simulink model "QD2_DroneStack_PID_FreqSwp_2021a"  (R2026a)
settings: Solver=ode1  StopTime=inf  FixedStep=1/1000  EnableMultiTasking=on
InitFcn:
  | Motor_Mapping_7_Inch
model workspace (MAT data in the model file):
  target_system = 1
undefined symbols (not defined in the file): _Commander, _Stabilizer, _SYSID, datetime, HIL, KT, lf, log_, log_QD2_, m, Motor_Matrix, n, qc_get_step_size, s, saved_data
libraries: quarc_library x107, simulink x30, simulink_extras x3, sl_discontinuities x2
(part 3 of 5)

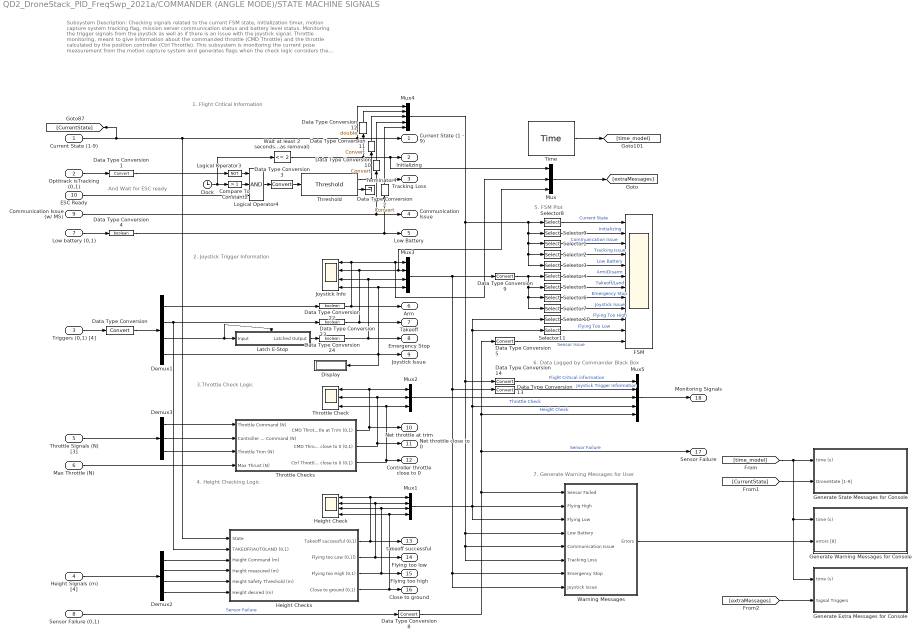
== system QD2_DroneStack_PID_FreqSwp_2021a/COMMANDER (ANGLE MODE)/STATE MACHINE SIGNALS ==
  note: 4. Height Checking Logic
  note: 3.Throttle Check Logic
  note: 2. Joystick Trigger Information
  note: 1. Flight Critical Information
  note: 6. Data Logged by Commander Black Box
  note: 5. FSM Plot
  note: 7. Generate Warning Messages for User
  note: Subsystem Description:
      | Checking signals related to the current FSM state, initialization timer, motion capture system tracking flag, mission server communication status and battery level status.
      | Monitoring the trigger signals from the joystick as well as if there is an issue with the joystick signal.
      | Throttle monitoring, meant to give information about the commanded throttle (CMD Throttle) and the throttle calculated by the position controller (Ctrl Throttle).
      | This subsystem is monitoring the current pose measurement from the motion capture system and generates flags when the check logic considers the QDrone flying to close to ground, too high or too low as well as generate a successful take off flag.
      | A subset of the FSM monitoring signals are shown using this scope. These signals are what Quanser considers importnat for flight.
      | FSM signals sent to the blackbox for post flight monitoring.
      | Error message generation based on flags generated by the FSM signal checks.
  note: And Wait for ESC ready
  Current State (1-9) : Inport
  "Optitrack isTracking (0,1)  " : Inport  Port=2
  Triggers (0,1) [4] : Inport  Port=3
  Height Signals (m) [4] : Inport  Port=4
  Throttle Signals (N) [3] : Inport  Port=5
  "Max Throttle (N) " : Inport  Port=6
  Low battery (0,1) : Inport  Port=7
  Sensor Failure (0,1) : Inport  Port=8
  Communication Issue (w/ MS) : Inport  Port=9
  ESC Ready : Inport  Port=10
  Clock : Clock
  Compare To Constant2 : simulink/Logic and Bit Operations/Compare To Constant  relop=>  const=1  OutDataTypeStr=boolean
  Data Type Conversion{,1..3,5,8..11,13..14} (11 alike) : DataTypeConversion  SaturateOnIntegerOverflow=off  RndMeth=Floor
  Data Type Conversion12 : DataTypeConversion  OutDataTypeStr=double  SaturateOnIntegerOverflow=off  RndMeth=Floor
  Data Type Conversion{4,22..24} (4 alike) : DataTypeConversion  OutDataTypeStr=boolean  SaturateOnIntegerOverflow=off  RndMeth=Floor
  Demux1 : Demux  Outputs=[1 1 1 1]
  Demux2 : Demux
  Demux3 : Demux  Outputs=3
  Display : Display
  FSM : Scope  NumInputPorts=12
      settings: TimeSpan=30  Title=Current State  ActiveDisplayYMinimum=0.9  ActiveDisplayYMaximum=1.1
  Generate Extra Messages for Console : Subsystem
  Generate State Messages for Console : Subsystem
  Generate Warning Messages for Console : Subsystem
  "Height Check " : Scope  NumInputPorts=4
      settings: Title=Takeoff Successful  ActiveDisplayYMinimum=-1  ActiveDisplayYMaximum=1  DataLoggingVariableName=ScopeData3
  Height Checks : Subsystem
  Joystick Info : Scope  NumInputPorts=4
      settings: Title=Arm
  Latch E-Stop : Subsystem  TreatAsAtomicUnit=on
  Logical Operator3 : Logic  Operator=NOT  AllPortsSameDT=off  OutDataTypeStr=boolean
  Logical Operator4 : Logic  Inputs=3  AllPortsSameDT=off  OutDataTypeStr=boolean
  Mux : Mux  Inputs=3
  Mux1 : Mux  Inputs=[1 1 1 1]
  Mux2 : Mux  Inputs=[1 1 1]
  Mux3 : Mux  Inputs=[1 1 1 1]
  Mux4 : Mux  Inputs=[1 1 1 1 1]
  Mux5 : Mux  Inputs=[5 4 3 4 1]
  Selector1 : Selector  InputPortWidth=5  IndexOptions=Index vector (dialog)  Indices=4  OutputSizes=1
  Selector10 : Selector  InputPortWidth=4  IndexOptions=Index vector (dialog)  Indices=3  OutputSizes=1
  Selector11 : Selector  InputPortWidth=4  IndexOptions=Index vector (dialog)  Indices=2  OutputSizes=1
  Selector2 : Selector  InputPortWidth=5  IndexOptions=Index vector (dialog)  Indices=3  OutputSizes=1
  Selector3 : Selector  InputPortWidth=5  IndexOptions=Index vector (dialog)  Indices=5  OutputSizes=1
  Selector4 : Selector  InputPortWidth=4  IndexOptions=Index vector (dialog)  Indices=1  OutputSizes=1
  Selector5 : Selector  InputPortWidth=4  IndexOptions=Index vector (dialog)  Indices=2  OutputSizes=1
  Selector6 : Selector  InputPortWidth=4  IndexOptions=Index vector (dialog)  Indices=3  OutputSizes=1
  Selector7 : Selector  InputPortWidth=4  IndexOptions=Index vector (dialog)  Indices=4  OutputSizes=1
  Selector8 : Selector  InputPortWidth=5  IndexOptions=Index vector (dialog)  Indices=1  OutputSizes=1
  Selector9 : Selector  InputPortWidth=5  IndexOptions=Index vector (dialog)  Indices=2  OutputSizes=1
  Terminator4 : Terminator
  Threshold : quarc_library/Discontinuities/Threshold  operator=>=  param_src=Specify via dialog  threshold=0.5  duration=0.2
      settings: SourceProductName=QUARC Targets
  Throttle Check : Scope  NumInputPorts=3
      settings: Title=Command Throttle At Trim  ActiveDisplayYMinimum=-0.125  ActiveDisplayYMaximum=1.125  DataLoggingVariableName=ScopeData2
  Throttle Checks : Subsystem
  Time : quarc_library/Sources/Time/Time  time_source=Wall clock  sample_time=qc_get_step_size
  "Wait at least 2 seconds to allow for initialization (e.g., bias removal)" : simulink/Logic and Bit Operations/Compare To Constant  relop=<=  const=2  OutDataTypeStr=boolean
  Warning Messages : Subsystem
  "Current State (1 - 9)  " : Outport  VectorParamsAs1DForOutWhenUnconnected=off
  Initializing : Outport  Port=2  VectorParamsAs1DForOutWhenUnconnected=off
  Tracking Loss : Outport  Port=3  VectorParamsAs1DForOutWhenUnconnected=off
  Communication Issue : Outport  Port=4  VectorParamsAs1DForOutWhenUnconnected=off
  Low Battery : Outport  Port=5  VectorParamsAs1DForOutWhenUnconnected=off
  Arm : Outport  Port=6  VectorParamsAs1DForOutWhenUnconnected=off
  Takeoff : Outport  Port=7  VectorParamsAs1DForOutWhenUnconnected=off
  Emergency Stop : Outport  Port=8  VectorParamsAs1DForOutWhenUnconnected=off
  "Joystick Issue " : Outport  Port=9  VectorParamsAs1DForOutWhenUnconnected=off
  Net throttle at trim : Outport  Port=10  VectorParamsAs1DForOutWhenUnconnected=off
  Net throttle close to 0 : Outport  Port=11  VectorParamsAs1DForOutWhenUnconnected=off
  Controller throttle close to 0 : Outport  Port=12  VectorParamsAs1DForOutWhenUnconnected=off
  takeoff successful : Outport  Port=13  VectorParamsAs1DForOutWhenUnconnected=off
  Flying too low : Outport  Port=14  VectorParamsAs1DForOutWhenUnconnected=off
  Flying too high : Outport  Port=15  VectorParamsAs1DForOutWhenUnconnected=off
  Close to ground : Outport  Port=16  VectorParamsAs1DForOutWhenUnconnected=off
  "  Sensor Failure" : Outport  Port=17  VectorParamsAs1DForOutWhenUnconnected=off
  Monitoring Signals : Outport  Port=18  VectorParamsAs1DForOutWhenUnconnected=off
  wires:
  ESC Ready/1 -> Logical Operator4/3
  [extraMessages] -> Generate Extra Messages for Console/2(Signal Triggers)
  Mux/1 -> [extraMessages]
  Warning Messages/1(Errors) -> Generate Warning Messages for Console/2(errors [8])
  [CurrentState] -> Generate State Messages for Console/2(DroneState [1-9])
  [time_model] -> Generate State Messages for Console/1(time (s)), Generate Extra Messages for Console/1(time (s)), Generate Warning Messages for Console/1(time (s))
  Time/1 -> [time_model]
  "Max Throttle (N) "/1 -> Throttle Checks/4(Max Thrust (N))
  "Wait at least 2 seconds to allow for initialization (e.g., bias removal)"/1 -> Initializing/1, Mux/1, Data Type Conversion12/1
  Data Type Conversion14/1 -> Mux5/1  "Flight Critical information"
  Data Type Conversion13/1 -> Mux5/2  "Joystick Trigger Information"
  Data Type Conversion12/1 -> Mux4/2
  Data Type Conversion11/1 -> Mux4/3
  Data Type Conversion10/1 -> Mux4/4
  Data Type Conversion2/1 -> Mux4/5
  Selector8/1 -> FSM/1  "Current State"
  Current State (1-9)/1 -> "Current State (1 - 9)  "/1, Mux4/1, Height Checks/1(State), [CurrentState]
  Data Type Conversion8/1 -> Warning Messages/1(Sensor Failed), Mux5/5, Data Type Conversion5/1, "  Sensor Failure"/1  "Sensor Failure"
  Data Type Conversion9/1 -> Selector6/1, Selector7/1, Selector5/1, Selector4/1
  Throttle Checks/3(Ctrl Throttle close to 0 (0,1)) -> Controller throttle close to 0/1, Throttle Check/3, Mux2/3
  Mux4/1 -> Selector8/1, Selector9/1, Selector1/1, Selector2/1, Selector3/1, Data Type Conversion14/1, Warning Messages/6(Tracking Loss), Warning Messages/5(Communication Issue), Warning Messages/4(Low Battery)
  Mux3/1 -> Data Type Conversion13/1, Warning Messages/8(Joystick Issue), Warning Messages/7("Emergency Stop "), Data Type Conversion9/1
  Mux2/1 -> Mux5/3  "Throttle Check"
  Mux1/1 -> Mux5/4, Selector10/1, Selector11/1, Warning Messages/2(Flying High), Warning Messages/3(Flying Low)  "Height Check"
  Mux5/1 -> Monitoring Signals/1
  Threshold/1 -> Tracking Loss/1, Data Type Conversion11/1
  Communication Issue (w/ MS)/1 -> Communication Issue/1, Data Type Conversion10/1
  Demux1/4 -> "Joystick Issue "/1, Mux3/4, Joystick Info/4, Display/1
  Data Type Conversion4/1 -> Low Battery/1, Data Type Conversion2/1
  Data Type Conversion22/1 -> Arm/1, Mux3/1, Mux/2, Joystick Info/1
  Data Type Conversion23/1 -> Takeoff/1, Mux3/2, Mux/3, Joystick Info/2
  Data Type Conversion24/1 -> Emergency Stop/1, Mux3/3, Joystick Info/3
  Selector11/1 -> FSM/11  "Flying Too Low"
  Selector10/1 -> FSM/10  "Flying Too High"
  Data Type Conversion5/1 -> FSM/12  "Sensor Issue"
  Selector7/1 -> FSM/9  "Joystick Issue"
  Selector6/1 -> FSM/8  "Emergency Stop"
  Selector5/1 -> FSM/7  "Takeoff/Land"
  Selector4/1 -> FSM/6  "Arm/Disarm"
  Selector3/1 -> FSM/5  "Low Battery"
  Selector2/1 -> FSM/4  "Tracking Issue"
  Selector1/1 -> FSM/3  "Communication Issue"
  Selector9/1 -> FSM/2  "Initializing"
  Demux1/3 -> Latch E-Stop/Trigger, Latch E-Stop/1(Input)
  Latch E-Stop/1(Latched Output) -> Data Type Conversion24/1
  "Optitrack isTracking (0,1)  "/1 -> Data Type Conversion1/1
  Logical Operator3/1 -> Logical Operator4/1
  Threshold/2 -> Terminator4/1
  Logical Operator4/1 -> Data Type Conversion3/1
  Clock/1 -> Compare To Constant2/1, "Wait at least 2 seconds to allow for initialization (e.g., bias removal)"/1
  Compare To Constant2/1 -> Logical Operator4/2
  Data Type Conversion3/1 -> Threshold/1
  Data Type Conversion1/1 -> Logical Operator3/1
  Sensor Failure (0,1)/1 -> Data Type Conversion8/1  "Sensor Failure"
  Height Checks/2(Flying too Low (0,1l)) -> "Height Check "/2, Mux1/2, Flying too low/1
  Low battery (0,1)/1 -> Data Type Conversion4/1
  Data Type Conversion/1 -> Demux1/1
  Height Checks/4(Close to ground (0,1)) -> Close to ground/1, Mux1/4, "Height Check "/4
  Height Checks/3(Flying too High (0,1)) -> Flying too high/1, "Height Check "/3, Mux1/3
  Throttle Checks/1(CMD Throttle at Trim (0,1)) -> Throttle Check/1, Mux2/1, Net throttle at trim/1
  Demux3/3 -> Throttle Checks/3(Throttle Trim (N))
  Demux3/2 -> Throttle Checks/2(Controller Throttle Command (N))
  Demux2/2 -> Height Checks/4(Height measured (m))
  Demux1/2 -> Height Checks/2(TAKEOFF/AUTOLAND (0,1)), Data Type Conversion23/1
  Demux2/3 -> Height Checks/5(Height Safety Threshold (m))
  Height Checks/1(Takeoff successful (0,1)) -> Mux1/1, "Height Check "/1, takeoff successful/1
  Throttle Checks/2(CMD Throttle close to 0 (0,1)) -> Net throttle close to 0/1, Throttle Check/2, Mux2/2
  Demux1/1 -> Data Type Conversion22/1
  Throttle Signals (N) [3]/1 -> Demux3/1
  Demux2/4 -> Height Checks/6(Height desired (m))
  Height Signals (m) [4]/1 -> Demux2/1
  Demux3/1 -> Throttle Checks/1(Throttle Command (N))
  Demux2/1 -> Height Checks/3(Height Command (m))
  Triggers (0,1) [4]/1 -> Data Type Conversion/1

== system QD2_DroneStack_PID_FreqSwp_2021a/COMMANDER (ANGLE MODE)/Signal Smoothing ==
  "High Frequency Controller Commands (N,rad, rad/s)[4]" : Inport
  Constant4 : Constant
  Constant5 : Constant  Value=100
  Mux : Mux  Inputs=2
  Second-Order Low-Pass Filter : quarc_library/Continuous/Second-Order Low-Pass Filter  params_source=External (input ports)  input_width=60  input_zeta=1  input_init=0
  Selector1 : Selector  InputPortWidth=4  IndexOptions=Index vector (dialog)  Indices=[3:4]  OutputSizes=1
  Selector3 : Selector  InputPortWidth=4  IndexOptions=Index vector (dialog)  Indices=[1:2]  OutputSizes=1
  Terminator : Terminator
  "Smoothed Controller Commands (N,rad, rad/s)[4]" : Outport
  wires:
  Second-Order Low-Pass Filter/2 -> Terminator/1
  Constant5/1 -> Second-Order Low-Pass Filter/2
  Constant4/1 -> Second-Order Low-Pass Filter/3
  Selector3/1 -> Second-Order Low-Pass Filter/1, Second-Order Low-Pass Filter/4
  Second-Order Low-Pass Filter/1 -> Mux/1
  Selector1/1 -> Mux/2
  Mux/1 -> "Smoothed Controller Commands (N,rad, rad/s)[4]"/1
  "High Frequency Controller Commands (N,rad, rad/s)[4]"/1 -> Selector3/1, Selector1/1

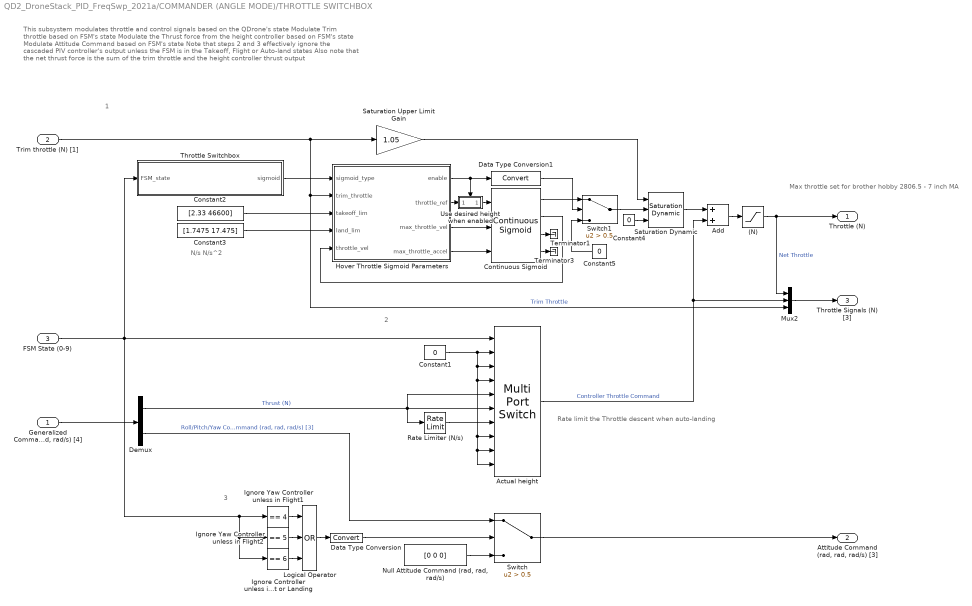
== system QD2_DroneStack_PID_FreqSwp_2021a/COMMANDER (ANGLE MODE)/THROTTLE SWITCHBOX  ==
  note: N/s N/s^2
  note: This subsystem modulates throttle and control signals based on the QDrone's state
      | Modulate Trim throttle based on FSM's state
      | Modulate the Thrust force from the height controller based on FSM's state
      | Modulate Attitude Command based on FSM's state
      |
      | Note that steps 2 and 3 effectively ignore the cascaded PIV controller's output unless the FSM is in the Takeoff, Flight or Auto-land states
      | Also note that the net thrust force is the sum of the trim throttle and the height controller thrust output
  note: Rate limit the Throttle descent when auto-landing
  note: 1
  note: 2
  note: 3
  note: Max throttle set for brother hobby 2806.5 - 7 inch MA
  "Generalized Command (N, rad, rad, rad/s) [4]" : Inport
  Trim throttle (N) [1] : Inport  Port=2
  FSM State (0-9) : Inport  Port=3
  (N) : Saturate  UpperLimit=58  LowerLimit=0
  Actual height : MultiPortSwitch  Inputs=9  SaturateOnIntegerOverflow=off  InputSameDT=off
  Add : Sum
  Constant1 : Constant  Value=0
  Constant2 : Constant  Value=[2.33 46600]
  Constant3 : Constant  Value=[1.7475 17.475]
  Constant4 : Constant  Value=0
  Constant5 : Constant  Value=0
  Continuous Sigmoid : quarc_library/Sources/Sigmoids/Continuous Sigmoid  params_source=External (input ports)  max_velocity=2  max_acceleration=10  initial_position=0  initial_velocity=0  hold_off=0.5  input_sample_time=-1  output_sample_time=qc_get_step_size
      settings: SourceProductName=QUARC Targets
  Data Type Conversion : DataTypeConversion  SaturateOnIntegerOverflow=off  RndMeth=Floor
  Data Type Conversion1 : DataTypeConversion  SaturateOnIntegerOverflow=off  RndMeth=Floor
  Demux : Demux  Outputs=[1 3]
  Hover Throttle Sigmoid Parameters : MATLAB Function  TreatAsAtomicUnit=on
  "Ignore Controller unless in Takeoff, Flight or Landing" : simulink/Logic and Bit Operations/Compare To Constant  relop===  const=6  OutDataTypeStr=boolean
  Ignore Yaw Controller unless in Flight1 : simulink/Logic and Bit Operations/Compare To Constant  relop===  const=4  OutDataTypeStr=boolean
  Ignore Yaw Controller unless in Flight2 : simulink/Logic and Bit Operations/Compare To Constant  relop===  const=5  OutDataTypeStr=boolean
  Logical Operator : Logic  Operator=OR  Inputs=3  AllPortsSameDT=off  OutDataTypeStr=boolean
  Mux2 : Mux  Inputs=3
  "Null Attitude Command (rad, rad, rad/s)" : Constant  Value=[0 0 0]
  Rate Limiter (N/s) : RateLimiter  RisingSlewLimit=100  FallingSlewLimit=-100  SampleTimeMode=inherited
  Saturation Dynamic : sl_discontinuities/Saturation Dynamic  OutMin=[]  OutMax=[]  OutDataTypeStr=Inherit: Same as second input  OutDataType=fixdt(1, 16)  OutScaling=2^-10  DoSatur=off
  Saturation Upper Limit Gain : Gain  Gain=1.05
  Switch : Switch  Criteria=u2 > Threshold  Threshold=0.5  SaturateOnIntegerOverflow=off  InputSameDT=off
  Switch1 : Switch  Criteria=u2 > Threshold  Threshold=0.5  SaturateOnIntegerOverflow=off  InputSameDT=off
  Terminator1 : Terminator
  Terminator3 : Terminator
  Throttle Switchbox : MATLAB Function  TreatAsAtomicUnit=on
  Use desired height when enabled : Subsystem  TreatAsAtomicUnit=on
  Throttle (N) : Outport  VectorParamsAs1DForOutWhenUnconnected=off
  "Attitude Command (rad, rad, rad/s) [3]" : Outport  Port=2  VectorParamsAs1DForOutWhenUnconnected=off
  Throttle Signals (N) [3] : Outport  Port=3  VectorParamsAs1DForOutWhenUnconnected=off
  wires:
  Rate Limiter (N/s)/1 -> Actual height/7
  Constant1/1 -> Actual height/2, Actual height/3, Actual height/4, Actual height/9, Actual height/10, Actual height/8
  Switch/1 -> "Attitude Command (rad, rad, rad/s) [3]"/1
  Constant5/1 -> Switch1/3
  Hover Throttle Sigmoid Parameters/2(throttle_ref) -> Use desired height when enabled/1(h_d (m) [1])
  Use desired height when enabled/1(Out1) -> Continuous Sigmoid/1
  Continuous Sigmoid/3 -> Terminator1/1
  Hover Throttle Sigmoid Parameters/1(enable) -> Use desired height when enabled/Enable, Data Type Conversion1/1
  Data Type Conversion1/1 -> Switch1/2
  Hover Throttle Sigmoid Parameters/3(max_throttle_vel) -> Continuous Sigmoid/2
  Continuous Sigmoid/4 -> Terminator3/1
  Continuous Sigmoid/1 -> Switch1/1
  Hover Throttle Sigmoid Parameters/4(max_throttle_accel) -> Continuous Sigmoid/3
  Constant2/1 -> Hover Throttle Sigmoid Parameters/3(takeoff_lim)
  Saturation Upper Limit Gain/1 -> Saturation Dynamic/1
  Throttle Switchbox/1(sigmoid) -> Hover Throttle Sigmoid Parameters/1(sigmoid_type)
  Trim throttle (N) [1]/1 -> Saturation Upper Limit Gain/1, Hover Throttle Sigmoid Parameters/2(trim_throttle), Mux2/3  "Trim Throttle"
  Switch1/1 -> Saturation Dynamic/2
  Constant3/1 -> Hover Throttle Sigmoid Parameters/4(land_lim)
  Saturation Dynamic/1 -> Add/1
  Constant4/1 -> Saturation Dynamic/3
  Continuous Sigmoid/2 -> Hover Throttle Sigmoid Parameters/5(throttle_vel)
  Demux/1 -> Actual height/5, Rate Limiter (N/s)/1, Actual height/6  "Thrust (N)"
  Logical Operator/1 -> Data Type Conversion/1
  "Ignore Controller unless in Takeoff, Flight or Landing"/1 -> Logical Operator/3
  FSM State (0-9)/1 -> Throttle Switchbox/1(FSM_state), Ignore Yaw Controller unless in Flight1/1, Ignore Yaw Controller unless in Flight2/1, "Ignore Controller unless in Takeoff, Flight or Landing"/1, Actual height/1
  Demux/2 -> Switch/1  "Roll/Pitch/Yaw Command (rad, rad, rad/s) [3]"
  Ignore Yaw Controller unless in Flight1/1 -> Logical Operator/1
  "Null Attitude Command (rad, rad, rad/s)"/1 -> Switch/3
  Data Type Conversion/1 -> Switch/2
  Ignore Yaw Controller unless in Flight2/1 -> Logical Operator/2
  Mux2/1 -> Throttle Signals (N) [3]/1
  "Generalized Command (N, rad, rad, rad/s) [4]"/1 -> Demux/1
  (N)/1 -> Throttle (N)/1, Mux2/1  "Net Throttle"
  Add/1 -> (N)/1
  Actual height/1 -> Add/2, Mux2/2  "Controller Throttle Command"

== system QD2_DroneStack_PID_FreqSwp_2021a/Communication/Detect Communication Loss ==
  note: Stream Loss: Check if the state is 2 and error is positive (error codes are negative). Otherwise issue a communication error.
      | OR
      | Data Loss: Check if the data is stale for a while (this is required because a connected stream may publish no new data). If stale, issue a communication error.
  State : Inport
  Error : Inport  Port=2
  Data Out : Inport  Port=3
  Clock1 : Clock
  Communication Loss : Scope  NumInputPorts=2
      settings: Title=Stream Loss  ActiveDisplayYMinimum=-0.1  ActiveDisplayYMaximum=1.1
  Data Type Conversion4 : DataTypeConversion  SaturateOnIntegerOverflow=off  RndMeth=Floor
  Grab mission server time to detect flat lines : Selector  InputPortWidth=17  IndexOptions=Index vector (dialog)  Indices=[16]  OutputSizes=1
  Logical Operator4 : Logic  Operator=OR  AllPortsSameDT=off  OutDataTypeStr=boolean
  MATLAB Function : MATLAB Function  TreatAsAtomicUnit=on
  Terminator3 : Terminator
  Terminator5 : Terminator
  Threshold1 : quarc_library/Discontinuities/Threshold  operator=>=  param_src=Specify via dialog  threshold=0.5  duration=0.1
      settings: SourceProductName=QUARC Targets
  Threshold2 : quarc_library/Discontinuities/Threshold  operator=>=  param_src=Specify via dialog  threshold=0.5  duration=0.5
      settings: SourceProductName=QUARC Targets
  Communication Issue : Outport  VectorParamsAs1DForOutWhenUnconnected=off
  wires:
  Threshold2/1 -> Communication Loss/2, Logical Operator4/2
  Logical Operator4/1 -> Data Type Conversion4/1
  Threshold1/2 -> Terminator3/1
  MATLAB Function/2(data_loss) -> Threshold2/1
  MATLAB Function/1(stream_connection_loss) -> Threshold1/1
  Clock1/1 -> MATLAB Function/1(time)
  Threshold2/2 -> Terminator5/1
  Threshold1/1 -> Communication Loss/1, Logical Operator4/1
  Grab mission server time to detect flat lines/1 -> MATLAB Function/4(ms_time)
  Data Out/1 -> Grab mission server time to detect flat lines/1
  State/1 -> MATLAB Function/2(state)
  Error/1 -> MATLAB Function/3(error)
  Data Type Conversion4/1 -> Communication Issue/1

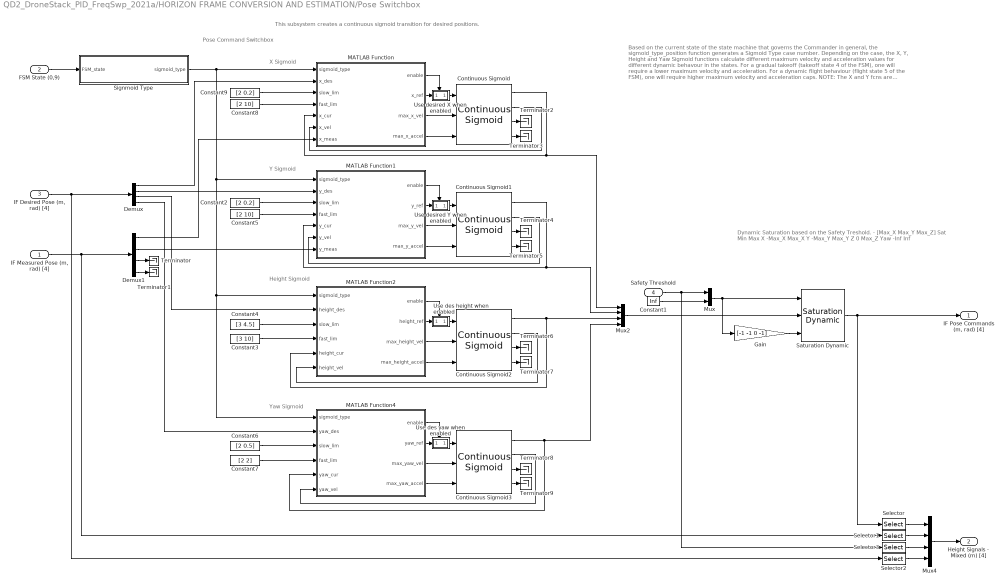
== system QD2_DroneStack_PID_FreqSwp_2021a/HORIZON FRAME CONVERSION AND ESTIMATION/Pose Switchbox ==
  note: Dynamic Saturation based on the Safety Treshold. - [Max_X Max_Y Max_Z]
      |
      | Sat Min Max
      | X -Max_X Max_X
      | Y -Max_Y Max_Y
      | Z 0 Max_Z
      | Yaw -Inf Inf
  note: Based on the current state of the state machine that governs the Commander in general,
      | the sigmoid_type_position function generates a Sigmoid Type case number. Depending on
      | the case, the X, Y, Height and Yaw Sigmoid functions calculate different maximum velocity
      | and acceleration values for different dynamic behavour in the states.
      |
      | For a gradual takeoff (takeoff state 4 of the FSM), one will require a lower maximum velocity
      | and acceleration. For a dynamic flight behaviour (flight state 5 of the FSM), one will require
      | higher maximum velocity and acceleration caps.
      |
      | NOTE: The X and Y fcns are logically identical due to the generally symmetric X and Y behaviour.
      | The Z and Yaw fcns are different.
  note: This subsystem creates a continuous sigmoid transition for desired positions.
  note: Height Sigmoid
  note: Pose Command Switchbox
  note: X Sigmoid
  note: Yaw Sigmoid
  note: Y Sigmoid
  "IF Measured Pose (m, rad) [4]" : Inport
  FSM State (0,9) : Inport  Port=2
  "IF Desired Pose (m, rad) [4]" : Inport  Port=3
  Safety Threshold : Inport  Port=4
  Constant1 : Constant  Value=Inf
  Constant2 : Constant  Value=[2 0.2]
  Constant3 : Constant  Value=[3 10]
  Constant4 : Constant  Value=[3 4.5]
  Constant5 : Constant  Value=[2 10]
  Constant6 : Constant  Value=[2 0.5]
  Constant7 : Constant  Value=[2 2]
  Constant8 : Constant  Value=[2 10]
  Constant9 : Constant  Value=[2 0.2]
  Continuous Sigmoid{,1..3} (4 alike) : quarc_library/Sources/Sigmoids/Continuous Sigmoid  params_source=External (input ports)  max_velocity=2  max_acceleration=10  initial_position=0  initial_velocity=0  hold_off=0.5  input_sample_time=-1  output_sample_time=qc_get_step_size
      settings: SourceProductName=QUARC Targets
  Demux : Demux
  Demux1 : Demux
  Gain : Gain  Gain=[-1 -1 0 -1]
  MATLAB Function : MATLAB Function  TreatAsAtomicUnit=on
  MATLAB Function1 : MATLAB Function  TreatAsAtomicUnit=on
  MATLAB Function2 : MATLAB Function  TreatAsAtomicUnit=on
  MATLAB Function4 : MATLAB Function  TreatAsAtomicUnit=on
  Mux : Mux  Inputs=2
  Mux2 : Mux
  Mux4 : Mux
  Saturation Dynamic : sl_discontinuities/Saturation Dynamic  OutMin=[]  OutMax=[]  OutDataTypeStr=Inherit: Same as second input  OutDataType=fixdt(1, 16)  OutScaling=2^-10  DoSatur=off
  Selector : Selector  InputPortWidth=4  IndexOptions=Index vector (dialog)  Indices=[3]  OutputSizes=1
  Selector1 : Selector  InputPortWidth=4  IndexOptions=Index vector (dialog)  Indices=[3]  OutputSizes=1
  Selector2 : Selector  InputPortWidth=4  IndexOptions=Index vector (dialog)  Indices=[3]  OutputSizes=1
  Selector3 : Selector  InputPortWidth=3  IndexOptions=Index vector (dialog)  Indices=[3]  OutputSizes=1
  Signmoid Type : MATLAB Function  TreatAsAtomicUnit=on
  Terminator{,1..9} (10 alike) : Terminator
  Use des height when enabled : Subsystem  TreatAsAtomicUnit=on
  Use des yaw when enabled : Subsystem  TreatAsAtomicUnit=on
  Use desired X when enabled : Subsystem  TreatAsAtomicUnit=on
  Use desired Y when enabled : Subsystem  TreatAsAtomicUnit=on
  "IF Pose Commands (m, rad) [4]" : Outport  VectorParamsAs1DForOutWhenUnconnected=off
  Height Signals - Mixed (m) [4] : Outport  Port=2  VectorParamsAs1DForOutWhenUnconnected=off
  wires:
  Constant4/1 -> MATLAB Function2/3(slow_lim)
  Constant3/1 -> MATLAB Function2/4(fast_lim)
  Selector/1 -> Mux4/1
  Selector1/1 -> Mux4/2
  Selector2/1 -> Mux4/4
  Selector3/1 -> Mux4/3
  Safety Threshold/1 -> Mux/1, Selector3/1
  Mux/1 -> Saturation Dynamic/1, Gain/1
  Constant1/1 -> Mux/2
  Saturation Dynamic/1 -> "IF Pose Commands (m, rad) [4]"/1, Selector/1
  Mux2/1 -> Saturation Dynamic/2
  Mux4/1 -> Height Signals - Mixed (m) [4]/1
  Gain/1 -> Saturation Dynamic/3
  Demux/2 -> MATLAB Function1/2(y_des)
  Use desired Y when enabled/1(Out1) -> Continuous Sigmoid1/1
  Use desired X when enabled/1(Out1) -> Continuous Sigmoid/1
  MATLAB Function2/3(max_height_vel) -> Continuous Sigmoid2/2
  Continuous Sigmoid3/3 -> Terminator8/1
  Demux1/4 -> Terminator1/1
  MATLAB Function4/1(enable) -> Use des yaw when enabled/Enable
  Use des yaw when enabled/1(Out1) -> Continuous Sigmoid3/1
  Continuous Sigmoid1/2 -> MATLAB Function1/6(y_vel)
  Constant2/1 -> MATLAB Function1/3(slow_lim)
  Constant6/1 -> MATLAB Function4/3(slow_lim)
  Demux1/1 -> MATLAB Function/7(x_meas)
  MATLAB Function1/2(y_ref) -> Use desired Y when enabled/1(h_d (m) [1])
  Demux/3 -> MATLAB Function2/2(height_des)
  Constant7/1 -> MATLAB Function4/4(fast_lim)
  Continuous Sigmoid1/4 -> Terminator5/1
  MATLAB Function1/1(enable) -> Use desired Y when enabled/Enable
  Continuous Sigmoid2/4 -> Terminator7/1
  Demux1/3 -> Terminator/1
  Signmoid Type/1(sigmoid_type) -> MATLAB Function/1(sigmoid_type), MATLAB Function1/1(sigmoid_type), MATLAB Function2/1(sigmoid_type), MATLAB Function4/1(sigmoid_type)
  MATLAB Function/3(max_x_vel) -> Continuous Sigmoid/2
  MATLAB Function2/1(enable) -> Use des height when enabled/Enable
  Constant9/1 -> MATLAB Function/3(slow_lim)
  Continuous Sigmoid2/2 -> MATLAB Function2/6(height_vel)
  Continuous Sigmoid1/1 -> MATLAB Function1/5(y_cur), Mux2/2
  MATLAB Function4/4(max_yaw_accel) -> Continuous Sigmoid3/3
  Demux/1 -> MATLAB Function/2(x_des)
  MATLAB Function1/3(max_y_vel) -> Continuous Sigmoid1/2
  Continuous Sigmoid3/2 -> MATLAB Function4/6(yaw_vel)
  MATLAB Function2/2(height_ref) -> Use des height when enabled/1(h_d (m) [1])
  MATLAB Function/4(max_x_accel) -> Continuous Sigmoid/3
  Use des height when enabled/1(Out1) -> Continuous Sigmoid2/1
  Continuous Sigmoid2/3 -> Terminator6/1
  Demux/4 -> MATLAB Function4/2(yaw_des)
  MATLAB Function1/4(max_y_accel) -> Continuous Sigmoid1/3
  MATLAB Function/1(enable) -> Use desired X when enabled/Enable
  Continuous Sigmoid3/4 -> Terminator9/1
  MATLAB Function4/2(yaw_ref) -> Use des yaw when enabled/1(h_d (m) [1])
  FSM State (0,9)/1 -> Signmoid Type/1(FSM_state)
  MATLAB Function2/4(max_height_accel) -> Continuous Sigmoid2/3
  Continuous Sigmoid/4 -> Terminator3/1
  Continuous Sigmoid/3 -> Terminator2/1
  Continuous Sigmoid/1 -> MATLAB Function/5(x_cur), Mux2/1
  Continuous Sigmoid/2 -> MATLAB Function/6(x_vel)
  MATLAB Function/2(x_ref) -> Use desired X when enabled/1(h_d (m) [1])
  Continuous Sigmoid3/1 -> MATLAB Function4/5(yaw_cur), Mux2/4
  MATLAB Function4/3(max_yaw_vel) -> Continuous Sigmoid3/2
  Continuous Sigmoid2/1 -> MATLAB Function2/5(height_cur), Mux2/3
  Demux1/2 -> MATLAB Function1/7(y_meas)
  Continuous Sigmoid1/3 -> Terminator4/1
  "IF Measured Pose (m, rad) [4]"/1 -> Demux1/1, Selector1/1
  "IF Desired Pose (m, rad) [4]"/1 -> Demux/1, Selector2/1
  Constant5/1 -> MATLAB Function1/4(fast_lim)
  Constant8/1 -> MATLAB Function/4(fast_lim)

== system QD2_DroneStack_PID_FreqSwp_2021a/QDrone 2 DAQ/Attitude Estimate from IMU Data ==
  IMU Data [12] : Inport
  For Each Subsystem - Iterate over IMU0 and IMU1 : Subsystem  TreatAsAtomicUnit=on
  Reshape into 2 columns for IMU0 and IMU1 : Reshape  OutputDimensionality=Customize  OutputDimensions=[6,2]
  Select Data for IMU0 : Selector  NumberOfDimensions=2  InputPortWidth=3  IndexOptions=Index vector (dialog),Index vector (dialog)  Indices=[1:9],[1]  OutputSizes=1,1
  Select Data for IMU1 : Selector  NumberOfDimensions=2  InputPortWidth=3  IndexOptions=Index vector (dialog),Index vector (dialog)  Indices=[1:9],[2]  OutputSizes=1,1
  "BF Estimated Attitude for IMU0 (rad, rad/s, rad/2^2) [9]" : Outport
  "BF Estimated Attitude for IMU1 (rad, rad/s, rad/2^2) [9]" : Outport  Port=2
  wires:
  Select Data for IMU1/1 -> "BF Estimated Attitude for IMU1 (rad, rad/s, rad/2^2) [9]"/1
  Select Data for IMU0/1 -> "BF Estimated Attitude for IMU0 (rad, rad/s, rad/2^2) [9]"/1
  For Each Subsystem - Iterate over IMU0 and IMU1/1("BF Estimated Attitude (rad, rad/s, rad/2^2) [9xn]") -> Select Data for IMU0/1, Select Data for IMU1/1
  Reshape into 2 columns for IMU0 and IMU1/1 -> For Each Subsystem - Iterate over IMU0 and IMU1/1(IMU Data [6xn])
  IMU Data [12]/1 -> Reshape into 2 columns for IMU0 and IMU1/1

== system QD2_DroneStack_PID_FreqSwp_2021a/QDrone 2 DAQ/Choose Motor Telemetry ==
  enable telemetry : Inport
  Bias1 : Bias  Bias=0:3  SaturateOnIntegerOverflow=off
  Constant1 : Constant  Value="[0 0 0 0; 1 0 0 0; 0 0 0 0; 0 1 0 0; 0 0 0 0; 0 0 1 0; 0 0 0 0;  0 0 0 1]"
  Constant2 : Constant  Value=8
  Gain : Gain  Gain=.7
  MATLAB Function : MATLAB Function  TreatAsAtomicUnit=on
  Selector : Selector  NumberOfDimensions=2  IndexMode=Zero-based  InputPortWidth=3  IndexOptions=Index vector (port),Select all  Indices=[1 3],1  OutputSizes=1,1
  Telemetry : Scope
      settings: TimeSpan=.02  ActiveDisplayYMinimum=-0.4625  ActiveDisplayYMaximum=4.1625  DataLoggingVariableName=ScopeData2
  Zero-Order Hold1 : ZeroOrderHold  SampleTime=-1
  Motor telemetry select : Outport
  Motor telemetry index : Outport  Port=2
  wires:
  Constant2/1 -> MATLAB Function/2(n)
  Constant1/1 -> Selector/1
  Selector/1 -> Gain/1, Motor telemetry select/1
  enable telemetry/1 -> MATLAB Function/1(enable)
  Zero-Order Hold1/1 -> Motor telemetry index/1, Selector/2
  MATLAB Function/1(idx) -> Zero-Order Hold1/1
  Bias1/1 -> Telemetry/1
  Gain/1 -> Bias1/1

== system QD2_DroneStack_PID_FreqSwp_2021a/QDrone 2 DAQ/Construct ESC Speed ==
  ESC Data In [4] : Inport
  ESC Channel Select : Inport  Port=2
  For Each Subsystem - Construct ESC Signal : Subsystem  TreatAsAtomicUnit=on
  Memory : Memory  InitialCondition=zeros(1,4)
  ESC Data Out [4] : Outport
  wires:
  ESC Channel Select/1 -> For Each Subsystem - Construct ESC Signal/2(ESC Channel)
  ESC Data In [4]/1 -> For Each Subsystem - Construct ESC Signal/1(ESC Data In [4])
  Memory/1 -> For Each Subsystem - Construct ESC Signal/3(ESC Previous Data [4])
  For Each Subsystem - Construct ESC Signal/1(ESC Data Out [4]) -> Memory/1, ESC Data Out [4]/1

== system QD2_DroneStack_PID_FreqSwp_2021a/QDrone 2 DAQ/Construct ESC Temperature ==
  ESC Data In [4] : Inport
  ESC Channel Select : Inport  Port=2
  For Each Subsystem - Construct ESC Signal : Subsystem  TreatAsAtomicUnit=on
  Memory : Memory  InitialCondition=zeros(1,4)
  ESC Data Out [4] : Outport
  wires:
  ESC Channel Select/1 -> For Each Subsystem - Construct ESC Signal/2(ESC Channel)
  ESC Data In [4]/1 -> For Each Subsystem - Construct ESC Signal/1(ESC Data In [4])
  Memory/1 -> For Each Subsystem - Construct ESC Signal/3(ESC Previous Data [4])
  For Each Subsystem - Construct ESC Signal/1(ESC Data Out [4]) -> Memory/1, ESC Data Out [4]/1

== system QD2_DroneStack_PID_FreqSwp_2021a/QDrone 2 DAQ/Construct ESC Voltage ==
  ESC Data In [4] : Inport
  ESC Channel Select : Inport  Port=2
  For Each Subsystem - Construct ESC Signal : Subsystem  TreatAsAtomicUnit=on
  Memory : Memory  InitialCondition=zeros(1,4)
  ESC Data Out [4] : Outport
  wires:
  For Each Subsystem - Construct ESC Signal/1(ESC Data Out [4]) -> ESC Data Out [4]/1, Memory/1
  Memory/1 -> For Each Subsystem - Construct ESC Signal/3(ESC Previous Data [4])
  ESC Data In [4]/1 -> For Each Subsystem - Construct ESC Signal/1(ESC Data In [4])
  ESC Channel Select/1 -> For Each Subsystem - Construct ESC Signal/2(ESC Channel)

== system QD2_DroneStack_PID_FreqSwp_2021a/QDrone 2 DAQ/Detect ESC Problems ==
  ESC Telemetry Enabled : Inport
  ESC Channel Request [4] : Inport  Port=2
  ESC Channel Reported [4] : Inport  Port=3
  AND : Logic  IconShape=distinctive  AllPortsSameDT=off  OutDataTypeStr=boolean
  Compare To Constant : simulink/Logic and Bit Operations/Compare To Constant  relop=>=  const=20  OutDataTypeStr=boolean
  Constant : Constant  Value=200
  Delay{,1..3} (4 alike) : Delay
  Demux{,1..2,8} (4 alike) : Demux
  ESC Channel Mismatrch : Scope  NumInputPorts=4
      settings: Title=Front Left (Motor 3)  ActiveDisplayYMinimum=-0.125  ActiveDisplayYMaximum=1.125  DataLoggingVariableName=ScopeData7
  ESC Channel Mismatrch Count : Scope  NumInputPorts=4
      settings: Title=Front Left (Motor 3)  ActiveDisplayYMinimum=-3.125  ActiveDisplayYMaximum=28.125  DataLoggingVariableName=ScopeData8
  ESC Channel Selection Index : Scope  NumInputPorts=4
      settings: Title=Front Left (Motor 3)  ActiveDisplayYMinimum=-0.125  ActiveDisplayYMaximum=1.125
  For Each Subsystem : Subsystem  TreatAsAtomicUnit=on
  MATLAB Function : MATLAB Function  TreatAsAtomicUnit=on
  Mux : Mux
  Mux{1..4} (4 alike) : Mux  Inputs=2
  ESC Comm Problem [4] : Outport
  wires:
  Mux1/1 -> ESC Channel Selection Index/4
  Mux2/1 -> ESC Channel Selection Index/3
  Mux3/1 -> ESC Channel Selection Index/2
  Mux4/1 -> ESC Channel Selection Index/1
  Demux2/4 -> Mux4/2
  Demux2/3 -> Mux3/2
  Demux2/2 -> Mux2/2
  Demux2/1 -> Mux1/2
  ESC Telemetry Enabled/1 -> AND/2
  Compare To Constant/1 -> ESC Comm Problem [4]/1
  MATLAB Function/1(n) -> Demux1/1, Compare To Constant/1
  Demux1/2 -> ESC Channel Mismatrch Count/3
  Demux1/1 -> ESC Channel Mismatrch Count/4
  Demux1/3 -> ESC Channel Mismatrch Count/2
  Demux1/4 -> ESC Channel Mismatrch Count/1
  Constant/1 -> MATLAB Function/2(buffer_size)
  Demux8/4 -> ESC Channel Mismatrch/1
  Demux8/3 -> ESC Channel Mismatrch/2
  Demux8/1 -> ESC Channel Mismatrch/4
  Demux8/2 -> ESC Channel Mismatrch/3
  AND/1 -> Demux8/1, MATLAB Function/1(u)
  For Each Subsystem/1(mismatched [4]) -> AND/1
  Mux/1 -> For Each Subsystem/1(Channel Requested [4])
  Delay/1 -> Mux/4, Mux4/1
  Delay1/1 -> Mux/3, Mux3/1
  Delay3/1 -> Mux1/1, Mux/1
  Delay2/1 -> Mux/2, Mux2/1
  ESC Channel Request [4]/1 -> Demux/1
  Demux/4 -> Delay/1
  Demux/3 -> Delay1/1
  Demux/2 -> Delay2/1
  Demux/1 -> Delay3/1
  ESC Channel Reported [4]/1 -> For Each Subsystem/2(Channel Reported [4]), Demux2/1

== system QD2_DroneStack_PID_FreqSwp_2021a/QDrone 2 DAQ/Enabled Subsystem - Write ESC Commands ==
  DShot Raw [4] : Inport
  Enable : EnablePort
  HIL Write PWM : quarc_library/Data Acquisition/Generic/Immediate I//O/HIL Write PWM  object_name=HIL-1  channels=[0:3]  sample_time=-1  active=off  vector_input=on  port_labels=channel numbers
      settings: AttributesFormatString=(%<object_name>)  SourceProductName=QUARC Targets
  wires:
  DShot Raw [4]/1 -> HIL Write PWM/1

== system QD2_DroneStack_PID_FreqSwp_2021a/QDrone 2 DAQ/Generate LED Pattern ==
  ESC States : Inport
  Blue Blue : Constant  Value=[0 0 1 0 0 1]
  Green Green : Constant  Value=[0 1 0 0 1 0]
  LED OFF : Constant  Value=[ 0 0 0 0 0 0]
  Multiport Switch : MultiPortSwitch  DataPortOrder=Specify indices  DataPortIndices={0,1,2,3,4,5,77,88,99}  DataPortForDefault=Additional data port  DiagnosticForDefault=Warning  SaturateOnIntegerOverflow=off  InputSameDT=off
  Red Blue : Constant  Value="[ 1 0 0 0 0 1   ]"
  Red Red : Constant  Value=[ 1 0 0 1 0 0]
  Red Yellow : Constant  Value="[ 1 0 0 1 1 0  ]"
  Yellow Blue : Constant  Value="[ 1 1 0 0 0 1  ]"
  Yellow Green : Constant  Value="[ 1 1 0 0 1 0  ]"
  Yellow Red : Constant  Value="[ 1 1 0 1 0 0  ]"
  Yellow Yellow : Constant  Value="[ 1 1 0 1 1 0  ]"
  LED Command : Outport
  wires:
  Red Yellow/1 -> Multiport Switch/6
  Yellow Red/1 -> Multiport Switch/5
  Yellow Green/1 -> Multiport Switch/3
  Green Green/1 -> Multiport Switch/7
  LED OFF/1 -> Multiport Switch/11
  Yellow Blue/1 -> Multiport Switch/8
  Red Blue/1 -> Multiport Switch/9
  Yellow Yellow/1 -> Multiport Switch/2
  Red Red/1 -> Multiport Switch/10
  Blue Blue/1 -> Multiport Switch/4
  ESC States/1 -> Multiport Switch/1
  Multiport Switch/1 -> LED Command/1

== system QD2_DroneStack_PID_FreqSwp_2021a/QDrone 2 DAQ/Monitor Battery Level ==
  note: Monitor Battery Level.
      | Flag Low Battery Error if
      | Battery level dips below
      | threshold for specified
      | threshold time period.
  Battery (V) : Inport
  AND : Logic  IconShape=distinctive  AllPortsSameDT=off  OutDataTypeStr=boolean
  Battery Low Time Threshold (s) : Constant  Value=0.3
  Constant : Constant  Value=0.5
  Data Type Conversion : DataTypeConversion  SaturateOnIntegerOverflow=off  RndMeth=Floor
  Data Type Conversion1 : DataTypeConversion  SaturateOnIntegerOverflow=off  RndMeth=Floor
  Greater than minimum expected voltage (Valid Battery Reading) : simulink/Logic and Bit Operations/Compare To Constant  relop=>  const=0.5  OutDataTypeStr=boolean
  Less than minimum threshold voltage (Battery level too low) : simulink/Logic and Bit Operations/Compare To Constant  relop=<=  const=14  OutDataTypeStr=boolean
  Terminator : Terminator
  Threshold : quarc_library/Discontinuities/Threshold  operator=>=  param_src=External input port  threshold=0  duration=0
      settings: SourceProductName=QUARC Targets
  Triggered Subsystem - Latching Flag : Subsystem  TreatAsAtomicUnit=on
  Low Battery : Outport
  wires:
  Data Type Conversion1/1 -> Low Battery/1
  Triggered Subsystem - Latching Flag/1(Out1) -> Data Type Conversion1/1
  Threshold/1 -> Triggered Subsystem - Latching Flag/Trigger
  Threshold/2 -> Terminator/1
  Data Type Conversion/1 -> Threshold/1
  Battery Low Time Threshold (s)/1 -> Threshold/3
  Constant/1 -> Threshold/2
  AND/1 -> Data Type Conversion/1
  Greater than minimum expected voltage (Valid Battery Reading)/1 -> AND/1
  Less than minimum threshold voltage (Battery level too low)/1 -> AND/2
  Battery (V)/1 -> Greater than minimum expected voltage (Valid Battery Reading)/1, Less than minimum threshold voltage (Battery level too low)/1

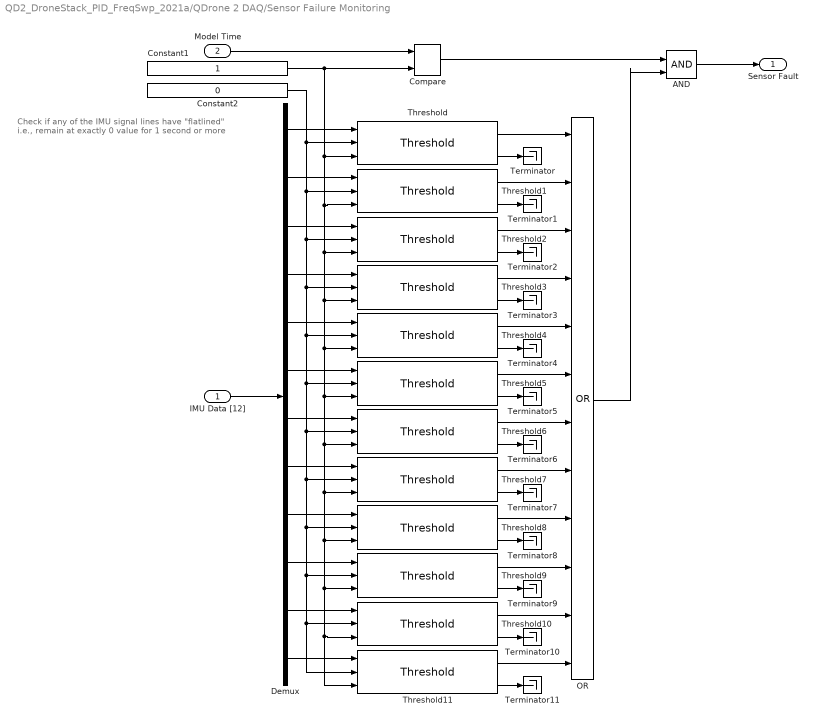
== system QD2_DroneStack_PID_FreqSwp_2021a/QDrone 2 DAQ/Sensor Failure Monitoring ==
  note: Check if any of the IMU signal lines have "flatlined"
      | i.e., remain at exactly 0 value for 1 second or more
  IMU Data [12] : Inport
  Model Time : Inport  Port=2
  AND : Logic  IconShape=distinctive  AllPortsSameDT=off  OutDataTypeStr=boolean
  Compare : quarc_library/Logic Operations/Compare  operator=>=  output_data_type=boolean
      settings: SourceProductName=QUARC Targets
  Constant1 : Constant
  Constant2 : Constant  Value=0
  Demux : Demux  Outputs=12
  OR : Logic  Operator=OR  Inputs=12  AllPortsSameDT=off  OutDataTypeStr=boolean
  Terminator{,1..11} (12 alike) : Terminator
  Threshold{,1..11} (12 alike) : quarc_library/Discontinuities/Threshold  operator===  param_src=External input port  threshold=0  duration=1
      settings: SourceProductName=QUARC Targets
  Sensor Fault : Outport
  wires:
  AND/1 -> Sensor Fault/1
  OR/1 -> AND/2
  Compare/1 -> AND/1
  Threshold11/2 -> Terminator11/1
  Threshold10/2 -> Terminator10/1
  Threshold9/2 -> Terminator9/1
  Threshold8/2 -> Terminator8/1
  Threshold7/2 -> Terminator7/1
  Threshold6/2 -> Terminator6/1
  Threshold5/2 -> Terminator5/1
  Threshold4/2 -> Terminator4/1
  Threshold3/2 -> Terminator3/1
  Threshold2/2 -> Terminator2/1
  Threshold1/2 -> Terminator1/1
  Threshold/2 -> Terminator/1
  Threshold11/1 -> OR/12
  Threshold10/1 -> OR/11
  Threshold9/1 -> OR/10
  Threshold8/1 -> OR/9
  Threshold7/1 -> OR/8
  Threshold6/1 -> OR/7
  Threshold5/1 -> OR/6
  Threshold4/1 -> OR/5
  Threshold3/1 -> OR/4
  Threshold2/1 -> OR/3
  Threshold1/1 -> OR/2
  Threshold/1 -> OR/1
  Demux/12 -> Threshold11/1
  Demux/11 -> Threshold10/1
  Demux/10 -> Threshold9/1
  Demux/9 -> Threshold8/1
  Demux/8 -> Threshold7/1
  Demux/7 -> Threshold6/1
  Demux/6 -> Threshold5/1
  Demux/5 -> Threshold4/1
  Demux/4 -> Threshold3/1
  Demux/3 -> Threshold2/1
  IMU Data [12]/1 -> Demux/1
  Constant2/1 -> Threshold/2, Threshold11/2, Threshold10/2, Threshold9/2, Threshold8/2, Threshold7/2, Threshold6/2, Threshold5/2, Threshold4/2, Threshold3/2, Threshold2/2, Threshold1/2
  Demux/2 -> Threshold1/1
  Demux/1 -> Threshold/1
  Constant1/1 -> Compare/2, Threshold/3, Threshold4/3, Threshold11/3, Threshold10/3, Threshold9/3, Threshold8/3, Threshold7/3, Threshold6/3, Threshold5/3, Threshold3/3, Threshold2/3, Threshold1/3
  Model Time/1 -> Compare/1

== system QD2_DroneStack_PID_FreqSwp_2021a/QDrone 2 DAQ/Timing Monitors ==
  note: ToF Range Rate (25 Hz)
  note: Optical Flow Rate (100 Hz)
  note: Base Model Rate (1kHz)
  Computation Time : quarc_library/Sources/Time/Computation Time  sample_time=qc_get_step_size  use_model=on  use_cpu_time=off
  Computation Time1 : quarc_library/Sources/Time/Computation Time  sample_time=0.01  use_model=on  use_cpu_time=off
  Computation Time2 : quarc_library/Sources/Time/Computation Time  sample_time=0.04  use_model=on  use_cpu_time=off
  Mux : Mux  Inputs=2
  Mux1 : Mux  Inputs=2
  Mux2 : Mux  Inputs=2
  Mux3 : Mux  Inputs=3
  Rate Transition{,1..3} (4 alike) : RateTransition
  Sample Time : quarc_library/Sources/Time/Sample Time  Priority=-99  sample_time=qc_get_step_size
  Sample Time1 : quarc_library/Sources/Time/Sample Time  Priority=-99  sample_time=0.01
  Sample Time2 : quarc_library/Sources/Time/Sample Time  Priority=-99  sample_time=0.04
  Timing Check : Scope  NumInputPorts=3
      settings: Title=Base Model Period (1ms)  ActiveDisplayYMinimum=-0.00162  ActiveDisplayYMaximum=0.01459  DataLoggingVariableName=ScopeData5
  Timings : Outport
  wires:
  Rate Transition3/1 -> Mux2/2
  Rate Transition2/1 -> Mux2/1
  Rate Transition1/1 -> Mux1/2
  Rate Transition/1 -> Mux1/1
  Mux3/1 -> Timings/1
  Mux2/1 -> Mux3/3, Timing Check/3
  Mux/1 -> Mux3/1, Timing Check/1
  Mux1/1 -> Timing Check/2, Mux3/2
  Sample Time2/1 -> Rate Transition3/1
  Computation Time2/1 -> Rate Transition2/1
  Computation Time1/1 -> Rate Transition/1
  Sample Time1/1 -> Rate Transition1/1
  Sample Time/1 -> Mux/2
  Computation Time/1 -> Mux/1

== system QD2_DroneStack_PID_FreqSwp_2021a/STABILIZER - QDRONE 2/FLIGHT SAFETY ==
  note: If the watchdog times out, stop the model. This will shut off the motors as well.
  note: If communication with the model supplying reference commands has been lost for some time while the drone is armed, stop the model. This will shut off the motors as well.
  note: If the model supplying reference commands triggers a STOP MODEL command, stop this model. This will shut off the motors as well.
  note: Log Computation Time. This must be less than 0.001 s
  note: Log Sample Time. This must be approximately 0.001 s
  note: Flight Safety Information
      |
      | When a warning/stop message pops up, this is the subsystem
      | that generates them.
      |
      | Monitor Sample/Computation Time
      | Stop this model
      | when Stop Model is generated
      | communication loss is detected
      | Also log the watchdog monitor output
  Arm : Inport
  Stop Model : Inport  Port=2
  Communication Loss : Inport  Port=3
  Communication : quarc_library/Discontinuities/Threshold  operator=>=  param_src=Specify via dialog  threshold=0.5  duration=1
      settings: SourceProductName=QUARC Targets
  Computation Time : quarc_library/Sources/Time/Computation Time  sample_time=qc_get_step_size  use_model=on  use_cpu_time=off
  Computation Time (s) : Scope
      settings: ActiveDisplayYMinimum=0.0004  ActiveDisplayYMaximum=0.0017  DataLoggingVariableName=ScopeData2
  Data Type Conversion1 : DataTypeConversion  SaturateOnIntegerOverflow=off  RndMeth=Floor
  Data Type Conversion3 : DataTypeConversion  OutDataTypeStr=double  SaturateOnIntegerOverflow=off  RndMeth=Floor
  Data Type Conversion4 : DataTypeConversion  SaturateOnIntegerOverflow=off  RndMeth=Floor
  Data Type Conversion5 : DataTypeConversion  SaturateOnIntegerOverflow=off  RndMeth=Floor
  HIL Watchdog : quarc_library/Data Acquisition/Generic/Watchdog/HIL Watchdog  object_name=HIL-1  timeout=0.1  sample_time=qc_get_step_size  active=off
      settings: AttributesFormatString=(%<object_name>)  SourceProductName=QUARC Targets
  Logical Operator1 : Logic  AllPortsSameDT=off  OutDataTypeStr=boolean
  Mux : Mux
  Mux1 : Mux  Inputs=2
  Sample Time : quarc_library/Sources/Time/Sample Time  Priority=-99  sample_time=qc_get_step_size
  Sample Time (s) : Scope
      settings: ActiveDisplayYMinimum=-0.00038  ActiveDisplayYMaximum=0.00212
  Stop model : quarc_library/Discontinuities/Threshold  operator=>=  param_src=Specify via dialog  threshold=0.5  duration=0.1
      settings: SourceProductName=QUARC Targets
  Stop with Message : quarc_library/Sinks/Error Handling/Stop with Message  message_type=Fixed error message  message_icon=Information  message=QDrone Stabilizer: Commander Terminated
  Stop with Message1 : quarc_library/Sinks/Error Handling/Stop with Message  message_type=Fixed error message  message_icon=Warning  message=QDrone Stabilizer: Communication with Commander lost
  Stop with Message3 : quarc_library/Sinks/Error Handling/Stop with Message  message_type=Fixed error message  message_icon=Information  message=QDrone Stabilizer: HIL Watchdog timer expired
  Terminator : Terminator
  Terminator1 : Terminator
  Safety Log : Outport  VectorParamsAs1DForOutWhenUnconnected=off
  wires:
  Data Type Conversion5/1 -> Mux/4
  Mux1/1 -> Mux/1
  Communication Loss/1 -> Logical Operator1/1
  Data Type Conversion3/1 -> Communication/1
  Communication/1 -> Stop with Message1/1, Data Type Conversion1/1
  Arm/1 -> Logical Operator1/2
  Data Type Conversion1/1 -> Mux/3
  Logical Operator1/1 -> Data Type Conversion3/1
  Communication/2 -> Terminator1/1
  Stop Model/1 -> Stop model/1
  Stop model/1 -> Stop with Message/1, Data Type Conversion4/1
  Stop model/2 -> Terminator/1
  HIL Watchdog/1 -> Data Type Conversion5/1, Stop with Message3/1
  Data Type Conversion4/1 -> Mux/2
  Sample Time/1 -> Mux1/1, Sample Time (s)/1
  Computation Time/1 -> Mux1/2, Computation Time (s)/1
  Mux/1 -> Safety Log/1

== system QD2_DroneStack_PID_FreqSwp_2021a/COMMANDER (ANGLE MODE)/STATE MACHINE SIGNALS/Generate Extra Messages for Console ==
  time (s) : Inport
  Signal Triggers : Inport  Port=2
  Boolean Edge-Based Triggered Print : Subsystem  TreatAsAtomicUnit=on
  Matrix Concatenate : Concatenate  NumInputs=3  Mode=Multidimensional array  ConcatenateDimension=2
  String Constant12 : quarc_library/Strings/String Constant  string_value=DRONE DISARMED  evaluate_string=off  string_type=text  max_length=80  sample_time=inf  variable_size=off
      settings: AttributesFormatString="\"DRONE DISARMED\""  SourceProductName=QUARC Targets
  String Constant13 : quarc_library/Strings/String Constant  string_value=DRONE LANDING  evaluate_string=off  string_type=text  max_length=80  sample_time=inf  variable_size=off
      settings: AttributesFormatString="\"DRONE LANDING\""  SourceProductName=QUARC Targets
  String Constant16 : quarc_library/Strings/String Constant  string_value=INITIALIZATION FINISHED  evaluate_string=off  string_type=text  max_length=80  sample_time=inf  variable_size=off
      settings: AttributesFormatString="\"INITIALIZATION FINISHED\""  SourceProductName=QUARC Targets
  Terminator : Terminator
  wires:
  Matrix Concatenate/1 -> Boolean Edge-Based Triggered Print/2(Message)
  time (s)/1 -> Boolean Edge-Based Triggered Print/3(time (s))
  Signal Triggers/1 -> Boolean Edge-Based Triggered Print/1(Signal Enable)
  String Constant16/1 -> Matrix Concatenate/1
  String Constant12/1 -> Matrix Concatenate/2
  String Constant13/1 -> Matrix Concatenate/3
  Boolean Edge-Based Triggered Print/1(Out1) -> Terminator/1
